simulink model "reactor_test10_sim"  (R2017b)
settings: Solver=ode23tb  StartTime=0.0  StopTime=tEndSimul  MaxStep=0.1  RelTol=5e-6
values from neighbouring files (symbols this model uses):
  c = conversion_factors()    [reactor_test10.m]
  dnDt = 0    [reactor_test10.m]
  h_heater_exterior = 10    [reactor_test10.m]
  h_heater_reactor = 1/R_heater_reactor    (= 400)    [reactor_test10.m]
  qOutIn = 100    [reactor_test10.m]
  Tamb_C = 25    [reactor_test10.m]
  tEnd_dnDt = 0    [reactor_test10.m]
  tEnd_Q = tStart_Q + 120 * c.min_to_sec    [reactor_test10.m]
  Tr_init = param.Tr_init    [reactor_test10.m]
  tStart_dnDt = 0    [reactor_test10.m]
  tStart_Q = 30 * c.min_to_sec    [reactor_test10.m]
undefined symbols (not defined in the file or in its folder): gas, h, liquid, NH3, P, T, T_heater_OFF_C, T_heater_ON_C, tEnd, tStart
libraries: thermochemical x17, simulink x3, dspsigops x1
settings Model: Creator=ferru  LastModifiedBy=fferrucc
settings SolverCC: AlgebraicLoopSolver=LineSearch

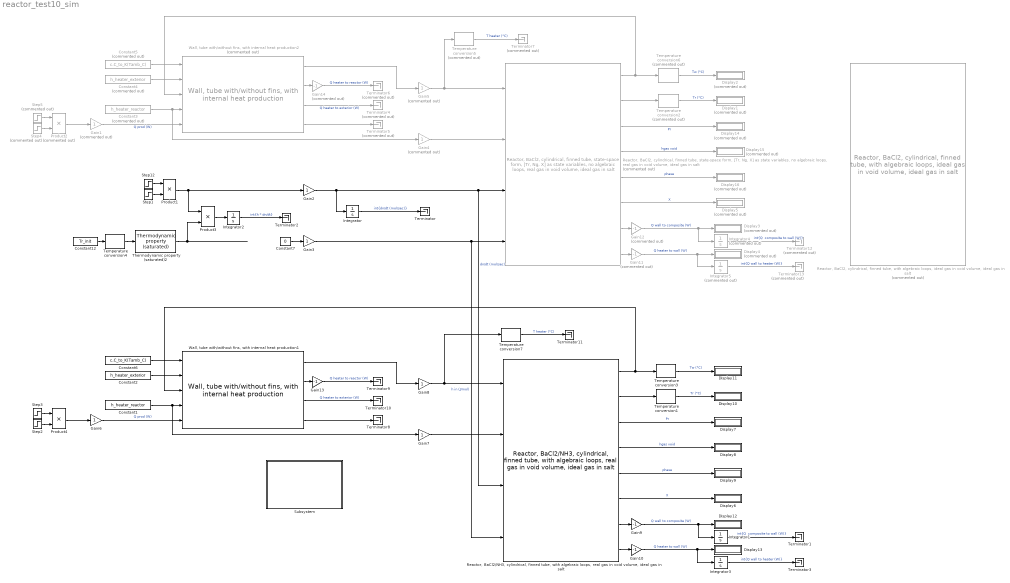
== system reactor_test10_sim ==
  Constant1 : Constant  Value=h_heater_reactor
  Constant12 : Constant  Value=Tr_init
  Constant2 : Constant  Value=h_heater_exterior
  Constant3 : Constant  Commented=on  Value=h_heater_reactor
  Constant4 : Constant  Commented=on  Value=h_heater_exterior
  Constant5 : Constant  Commented=on  Value=c.C_to_K(Tamb_C)
  Constant6 : Constant  Value=c.C_to_K(Tamb_C)
  Constant7 : Constant  Value=0
  Display{1..5,14..16} (8 alike) : Display  Commented=on
  Display{6..13} (8 alike) : Display
  Gain1 : Gain  Commented=on
  Gain10 : Gain  Gain=-1
  Gain11 : Gain  Commented=on  Gain=-1
  Gain12 : Gain  Commented=on  Gain=-1
  Gain13 : Gain  Gain=-1
  Gain14 : Gain  Commented=on  Gain=-1
  Gain{2..3,6..8} (5 alike) : Gain
  Gain4 : Gain  Commented=on
  Gain5 : Gain  Commented=on
  Gain9 : Gain  Gain=-1
  Integrator{,1..3} (4 alike) : Integrator
  Integrator4 : Integrator  Commented=on
  Integrator5 : Integrator  Commented=on
  Product1 : Product
  Product2 : Product  Commented=on
  Product3 : Product
  Product4 : Product
  "Reactor, BaCl2, cylindrical, finned tube, state-space form, [Tr, Ng, X] as state variables, no algebraic loops, real gas in void volume, ideal gas in salt" : thermochemical/Reactors/Reactor, BaCl2//NH3, state-space form, [Tr, Ng, X] as state variables, no algebraic loops, real gas in void volume, ideal gas in salt/Reactor, BaCl2, cylindrical, finned tube, state-space form, [Tr, Ng, X] as state variables, no algebraic loops, real gas in void volume, ideal gas in salt  Commented=on
      link override "Reactor, BaCl2//NH3, cylindrical, no walls, state-space form, [Tr, Ng, X] as state variables, no algebraic loops, real gas in void volume, ideal gas in salt": tao_salt=param.tao_salt  rho_composite=param.rho_composite  K_cin=K_cin  fluid=fluid  Lr=param.Lr  Lr_total=param.Lr_total  Dr=param.D  Ddiff=param.Ddiff  Tr_init=param.Tr_init  X_init=param.X_init
      link override "Wall, tube with//without fins": L_m=param.Lr_total  OD_mm=OD_mm  e_mm=thickness_mm  Tinit=Ttube_init
      settings: SourceProductName=@ Thermochemical
  "Reactor, BaCl2, cylindrical, finned tube, with algebraic loops, ideal gas in void volume, ideal gas in salt" : thermochemical/Reactors/Reactor, BaCl2//NH3, with algebraic loops, ideal gas in void volume, ideal gas in salt/Reactor, BaCl2, cylindrical, finned tube, with algebraic loops, ideal gas in void volume, ideal gas in salt  Commented=on
      link override "Reactor, BaCl2//NH3, cylindrical, no walls, with algebraic loops, ideal gas in void volume, ideal gas in salt": tao_salt=param.tao_salt  rho_composite=param.rho_composite  K_cin=K_cin  fluid=fluid  Lr=param.Lr  Lr_total=param.Lr_total  Dr=param.D  Ddiff=param.Ddiff  Tr_init=param.Tr_init  X_init=param.X_init
      link override "Wall, tube with//without fins": L_m=param.Lr_total  OD_mm=OD_mm  e_mm=thickness_mm  Tinit=Ttube_init
      settings: SourceProductName=@ Thermochemical
  "Reactor, BaCl2/NH3, cylindrical, finned tube, with algebraic loops, real gas in void volume, ideal gas in salt" : thermochemical/Reactors/Reactor, BaCl2//NH3, with algebraic loops, real gas in void volume, ideal gas in salt/Reactor, BaCl2//NH3, cylindrical, finned tube, with algebraic loops, real gas in void volume, ideal gas in salt
      link override "Reactor, BaCl2//NH3, cylindrical, no walls, with algebraic loops, real gas in void volume, ideal gas in salt": tao_salt=param.tao_salt  rho_composite=param.rho_composite  K_cin=K_cin  fluid=fluid  Lr=param.Lr  Lr_total=param.Lr_total  Dr=param.D  Ddiff=param.Ddiff  Tr_init=param.Tr_init  X_init=param.X_init
      link override "Wall, tube with//without fins": L_m=param.Lr_total  OD_mm=OD_mm  e_mm=thickness_mm  Tinit=Ttube_init
      settings: SourceProductName=@ Thermochemical
  Step1 : Step  Time=tEnd_dnDt  Before=1  After=0  SampleTime=0
  Step12 : Step  Time=tStart_dnDt  After=dnDt  SampleTime=0
  Step2 : Step  Time=tEnd_Q  Before=1  After=0  SampleTime=0
  Step3 : Step  Time=tStart_Q  After=qOutIn  SampleTime=0
  Step4 : Step  Commented=on  Time=tEnd_Q  Before=1  After=0  SampleTime=0
  Step5 : Step  Commented=on  Time=tStart_Q  After=qOutIn  SampleTime=0
  Subsystem : Subsystem
  Temperature conversion1 : thermochemical/Conversions/Temperature conversion  sel=K --> °C
      settings: SourceProductName=@ Thermochemical
  Temperature conversion2 : thermochemical/Conversions/Temperature conversion  Commented=on  sel=K --> °C
      settings: SourceProductName=@ Thermochemical
  Temperature conversion3 : thermochemical/Conversions/Temperature conversion  sel=K --> °C
      settings: SourceProductName=@ Thermochemical
  Temperature conversion4 : thermochemical/Conversions/Temperature conversion  sel=°C --> K
      settings: SourceProductName=@ Thermochemical
  Temperature conversion5 : thermochemical/Conversions/Temperature conversion  Commented=on  sel=K --> °C
      settings: SourceProductName=@ Thermochemical
  Temperature conversion6 : thermochemical/Conversions/Temperature conversion  Commented=on  sel=K --> °C
      settings: SourceProductName=@ Thermochemical
  Temperature conversion7 : thermochemical/Conversions/Temperature conversion  sel=K --> °C
      settings: SourceProductName=@ Thermochemical
  Terminator{,1..3,8..11} (8 alike) : Terminator
  Terminator{4..7,12..13} (6 alike) : Terminator  Commented=on
  Thermodynamic property (saturated)2 : thermochemical/Thermodynamic fluid properties/Thermodynamic  property (saturated)  sel=h(T) vap. (J/mol)  fluid=fluid  lookup1D_BreakPoint1=fluid.sat.T  lookup1D_Data=fluid.sat.vap.h_molar
      settings: SourceProductName=@ Thermochemical
  "Wall, tube with/without fins, with internal heat production1" : thermochemical/Walls/Wall, tube with//without fins, with internal heat production  L_m=heater_length_m  OD_mm=heater_OD_mm  e_mm=heater_thickness_mm  material_tube=Steel  cp_tube=464.5  rho_tube=7847  height_fin_mm=0  thickness_fin_mm=0  pitch_fin_mm=0  material_fin=Aluminum 1100  cp_fin=905.9  rho_fin=2658  lambda_fin=211.8  Tinit=Theater_init  mass_tube=2.829  mass_fin=0  mass_total=2.829  s_inner=0.35744  s_outer=0.3636
      settings: SourceProductName=@ Thermochemical
  "Wall, tube with/without fins, with internal heat production2" : thermochemical/Walls/Wall, tube with//without fins, with internal heat production  Commented=on  L_m=heater_length_m  OD_mm=heater_OD_mm  e_mm=heater_thickness_mm  material_tube=Steel  cp_tube=464.5  rho_tube=7847  height_fin_mm=0  thickness_fin_mm=0  pitch_fin_mm=0  material_fin=Aluminum 1100  cp_fin=905.9  rho_fin=2658  lambda_fin=211.8  Tinit=Theater_init  mass_tube=2.829  mass_fin=0  mass_total=2.829  s_inner=0.35744  s_outer=0.3636
      settings: SourceProductName=@ Thermochemical
  wires:
  Gain2/1 -> Integrator/1, "Reactor, BaCl2, cylindrical, finned tube, state-space form, [Tr, Ng, X] as state variables, no algebraic loops, real gas in void volume, ideal gas in salt"/3, "Reactor, BaCl2/NH3, cylindrical, finned tube, with algebraic loops, real gas in void volume, ideal gas in salt"/3  "dn/dt (mol/sec)"
  Gain3/1 -> "Reactor, BaCl2, cylindrical, finned tube, state-space form, [Tr, Ng, X] as state variables, no algebraic loops, real gas in void volume, ideal gas in salt"/4, "Reactor, BaCl2/NH3, cylindrical, finned tube, with algebraic loops, real gas in void volume, ideal gas in salt"/4  "h in (J/mol)"
  "Reactor, BaCl2/NH3, cylindrical, finned tube, with algebraic loops, real gas in void volume, ideal gas in salt"/3 -> Display7/1  "Pr"
  "Reactor, BaCl2/NH3, cylindrical, finned tube, with algebraic loops, real gas in void volume, ideal gas in salt"/4 -> Display8/1  "hgas void"
  "Reactor, BaCl2/NH3, cylindrical, finned tube, with algebraic loops, real gas in void volume, ideal gas in salt"/2 -> Temperature conversion1/1
  "Reactor, BaCl2/NH3, cylindrical, finned tube, with algebraic loops, real gas in void volume, ideal gas in salt"/6 -> Display6/1  "X"
  "Reactor, BaCl2/NH3, cylindrical, finned tube, with algebraic loops, real gas in void volume, ideal gas in salt"/5 -> Display9/1  "phase"
  Product1/1 -> Gain2/1, Product3/1
  Step12/1 -> Product1/1
  Step1/1 -> Product1/2
  Integrator/1 -> Terminator/1  "int{dn/dt (mol/sec)}"
  Integrator1/1 -> Terminator1/1  "int{Q  composite to wall (W)}"
  Temperature conversion1/1 -> Display10/1  "Tr (°C)"
  Constant12/1 -> Temperature conversion4/1
  Thermodynamic property (saturated)2/1 -> Product3/2
  Temperature conversion4/1 -> Thermodynamic property (saturated)2/1
  Integrator2/1 -> Terminator2/1  "int{h * dn/dt}"
  Product3/1 -> Integrator2/1
  Temperature conversion3/1 -> Display11/1  "Tw (°C)"
  "Reactor, BaCl2/NH3, cylindrical, finned tube, with algebraic loops, real gas in void volume, ideal gas in salt"/7 -> Gain9/1
  "Reactor, BaCl2/NH3, cylindrical, finned tube, with algebraic loops, real gas in void volume, ideal gas in salt"/8 -> Gain10/1
  Temperature conversion2/1 -> Display1/1  "Tr (°C)"
  Temperature conversion6/1 -> Display2/1  "Tw (°C)"
  "Reactor, BaCl2, cylindrical, finned tube, state-space form, [Tr, Ng, X] as state variables, no algebraic loops, real gas in void volume, ideal gas in salt"/4 -> Display15/1  "hgas void"
  "Reactor, BaCl2, cylindrical, finned tube, state-space form, [Tr, Ng, X] as state variables, no algebraic loops, real gas in void volume, ideal gas in salt"/5 -> Display16/1  "phase"
  "Reactor, BaCl2, cylindrical, finned tube, state-space form, [Tr, Ng, X] as state variables, no algebraic loops, real gas in void volume, ideal gas in salt"/2 -> Temperature conversion2/1
  "Reactor, BaCl2, cylindrical, finned tube, state-space form, [Tr, Ng, X] as state variables, no algebraic loops, real gas in void volume, ideal gas in salt"/6 -> Display5/1  "X"
  "Reactor, BaCl2, cylindrical, finned tube, state-space form, [Tr, Ng, X] as state variables, no algebraic loops, real gas in void volume, ideal gas in salt"/3 -> Display14/1  "Pr"
  Gain5/1 -> "Reactor, BaCl2, cylindrical, finned tube, state-space form, [Tr, Ng, X] as state variables, no algebraic loops, real gas in void volume, ideal gas in salt"/1, Temperature conversion5/1
  Gain4/1 -> "Reactor, BaCl2, cylindrical, finned tube, state-space form, [Tr, Ng, X] as state variables, no algebraic loops, real gas in void volume, ideal gas in salt"/2
  Integrator3/1 -> Terminator3/1  "int{Q wall to heater (W)}"
  Constant4/1 -> "Wall, tube with/without fins, with internal heat production2"/2
  Constant5/1 -> "Wall, tube with/without fins, with internal heat production2"/1
  Gain1/1 -> "Wall, tube with/without fins, with internal heat production2"/5  "Q prod (W)"
  Step4/1 -> Product2/2
  Step5/1 -> Product2/1
  Product2/1 -> Gain1/1
  Temperature conversion5/1 -> Terminator7/1  "T heater (°C)"
  "Wall, tube with/without fins, with internal heat production2"/1 -> Gain5/1
  Constant3/1 -> "Wall, tube with/without fins, with internal heat production2"/4, Gain4/1
  "Reactor, BaCl2, cylindrical, finned tube, state-space form, [Tr, Ng, X] as state variables, no algebraic loops, real gas in void volume, ideal gas in salt"/1 -> "Wall, tube with/without fins, with internal heat production2"/3, Temperature conversion6/1
  Temperature conversion7/1 -> Terminator11/1  "T heater (°C)"
  "Wall, tube with/without fins, with internal heat production1"/3 -> Terminator10/1  "Q heater to exterior (W)"
  Gain7/1 -> "Reactor, BaCl2/NH3, cylindrical, finned tube, with algebraic loops, real gas in void volume, ideal gas in salt"/2
  Product4/1 -> Gain6/1
  Constant1/1 -> Gain7/1, "Wall, tube with/without fins, with internal heat production1"/4
  "Reactor, BaCl2/NH3, cylindrical, finned tube, with algebraic loops, real gas in void volume, ideal gas in salt"/1 -> "Wall, tube with/without fins, with internal heat production1"/3, Temperature conversion3/1
  Constant2/1 -> "Wall, tube with/without fins, with internal heat production1"/2
  Gain6/1 -> "Wall, tube with/without fins, with internal heat production1"/5  "Q prod (W)"
  "Wall, tube with/without fins, with internal heat production1"/2 -> Gain13/1
  Step3/1 -> Product4/1
  Constant6/1 -> "Wall, tube with/without fins, with internal heat production1"/1
  "Wall, tube with/without fins, with internal heat production1"/4 -> Terminator8/1
  Step2/1 -> Product4/2
  "Wall, tube with/without fins, with internal heat production1"/1 -> Gain8/1
  Gain8/1 -> Temperature conversion7/1, "Reactor, BaCl2/NH3, cylindrical, finned tube, with algebraic loops, real gas in void volume, ideal gas in salt"/1
  Gain9/1 -> Integrator1/1, Display12/1  "Q wall to composite (W)"
  Gain10/1 -> Integrator3/1, Display13/1  "Q heater to wall (W)"
  Gain11/1 -> Integrator5/1, Display4/1  "Q heater to wall (W)"
  "Reactor, BaCl2, cylindrical, finned tube, state-space form, [Tr, Ng, X] as state variables, no algebraic loops, real gas in void volume, ideal gas in salt"/8 -> Gain11/1
  Integrator4/1 -> Terminator12/1  "int{Q  composite to wall (W)}"
  Gain12/1 -> Integrator4/1, Display3/1  "Q wall to composite (W)"
  Integrator5/1 -> Terminator13/1  "int{Q wall to heater (W)}"
  "Reactor, BaCl2, cylindrical, finned tube, state-space form, [Tr, Ng, X] as state variables, no algebraic loops, real gas in void volume, ideal gas in salt"/7 -> Gain12/1
  Gain13/1 -> Terminator9/1  "Q heater to reactor (W)"
  "Wall, tube with/without fins, with internal heat production2"/4 -> Terminator5/1
  "Wall, tube with/without fins, with internal heat production2"/3 -> Terminator4/1  "Q heater to exterior (W)"
  "Wall, tube with/without fins, with internal heat production2"/2 -> Gain14/1
  Gain14/1 -> Terminator6/1  "Q heater to reactor (W)"
  Constant7/1 -> Gain3/1

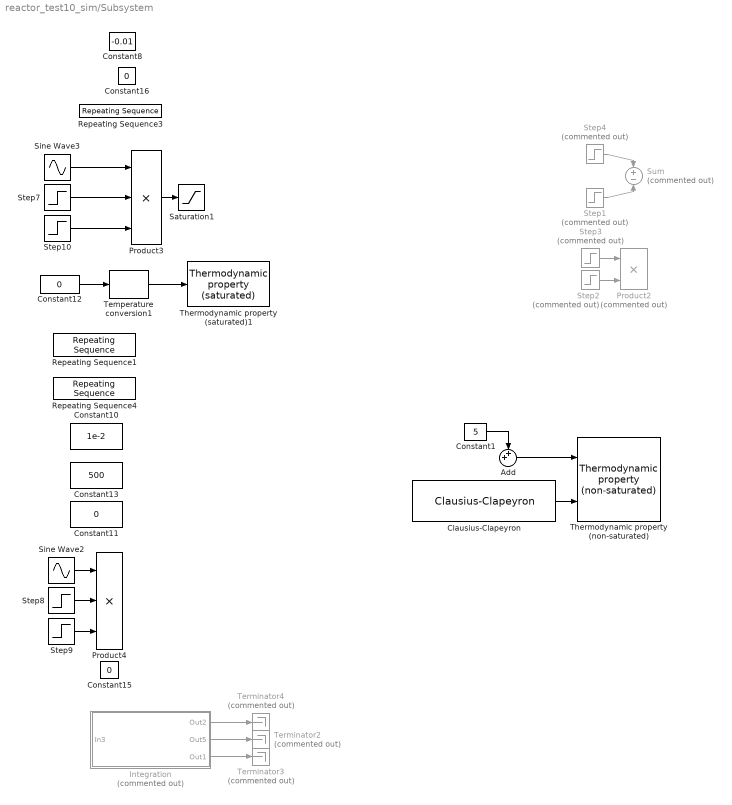
== system reactor_test10_sim/Subsystem ==
  Add : Sum  Inputs=++|
  Clausius-Clapeyron : thermochemical/Thermodynamic fluid properties/Clausius-Clapeyron  sel_1=P(T)  sel_2=NH3(liquid)/NH3(gas)
      settings: SourceProductName=@ Thermochemical
  Constant1 : Constant  Value=5
  Constant10 : Constant  Value=1e-2
  Constant{11..12,15..16} (4 alike) : Constant  Value=0
  Constant13 : Constant  Value=500
  Constant8 : Constant  Value=-0.01
  Integration : Subsystem  Commented=on  mask{T1=tStart, T2=tEnd}
      mask prompts: T1 "Integration time window, start time (sec)"; T2 "Integration time window, stop time (sec)"
  Product2 : Product  Commented=on
  Product3 : Product  Inputs=3
  Product4 : Product  Inputs=3
  Repeating Sequence1 : simulink/Sources/Repeating Sequence  rep_seq_t=[0, 100, 101, 200, 201]  rep_seq_y=[0, 0, 0.01, 0.01, 0]
  Repeating Sequence3 : simulink/Sources/Repeating Sequence  rep_seq_t=[0, 1, 1.001, 1.1, 1.1001, 1.2, 1.2002, 1.3, 1.3001]*1e3  rep_seq_y=[0, 0, 1, 1, 0, 0, 1, 1, 0]*(-0.01)
  Repeating Sequence4 : simulink/Sources/Repeating Sequence  rep_seq_t=[0, 99, 100, 199, 200 299]  rep_seq_y=1000*[0, 0, 1, 1, -1, -1]
  Saturation1 : Saturate  UpperLimit=Inf  LowerLimit=0
  Sine Wave2 : Sin  Amplitude=1e3  Frequency=2*pi/1e2  SampleTime=0
  Sine Wave3 : Sin  Amplitude=0.01  Bias=0.01  Frequency=2*pi/1e2  SampleTime=0
  Step1 : Step  Commented=on  Time=tEnd  After=T_heater_ON_C-T_heater_OFF_C  SampleTime=0
  Step10 : Step  Time=2e3  Before=1  After=0  SampleTime=0
  Step2 : Step  Commented=on  Time=tEnd  Before=1  After=0  SampleTime=0
  Step3 : Step  Commented=on  Time=tStart  After=qOutIn  SampleTime=0
  Step4 : Step  Commented=on  Time=tStart  Before=T_heater_OFF_C  After=T_heater_ON_C  SampleTime=0
  Step7 : Step  Time=1e3  SampleTime=0
  Step8 : Step  Time=1e3  SampleTime=0
  Step9 : Step  Time=2e3  Before=1  After=0  SampleTime=0
  Sum : Sum  Commented=on  Inputs=+-
  Temperature conversion1 : thermochemical/Conversions/Temperature conversion  sel=°R --> °F
      settings: SourceProductName=@ Thermochemical
  Terminator2 : Terminator  Commented=on
  Terminator3 : Terminator  Commented=on
  Terminator4 : Terminator  Commented=on
  Thermodynamic property (non-saturated) : thermochemical/Thermodynamic fluid properties/Thermodynamic  property (non-saturated)  sel=h(T,P)  fluid=fluid  reciprocVar=-1  lookup2D_BreakPoint1=fluid.no_sat.T_P_indep.var_indep.T  lookup2D_BreakPoint2=fluid.no_sat.T_P_indep.var_indep.P  lookup2D_Data=fluid.no_sat.T_P_indep.var_dep.h_molar
      settings: SourceProductName=@ Thermochemical
  Thermodynamic property (saturated)1 : thermochemical/Thermodynamic fluid properties/Thermodynamic  property (saturated)  sel=h(T) vap. (J/mol)  fluid=fluid  lookup1D_BreakPoint1=fluid.sat.T  lookup1D_Data=fluid.sat.vap.h_molar
      settings: SourceProductName=@ Thermochemical
  wires:
  Step7/1 -> Product3/2
  Product3/1 -> Saturation1/1
  Sine Wave2/1 -> Product4/1
  Sine Wave3/1 -> Product3/1
  Step8/1 -> Product4/2
  Step10/1 -> Product3/3
  Step9/1 -> Product4/3
  Temperature conversion1/1 -> Thermodynamic property (saturated)1/1
  Constant12/1 -> Temperature conversion1/1
  Integration/2(Out5) -> Terminator2/1
  Integration/3(Out1) -> Terminator3/1
  Integration/1(Out2) -> Terminator4/1
  Add/1 -> Thermodynamic property (non-saturated)/1
  Constant1/1 -> Add/1
  Clausius-Clapeyron/1 -> Thermodynamic property (non-saturated)/2
  ? -> Clausius-Clapeyron/1, Add/2
  Step3/1 -> Product2/1
  Step2/1 -> Product2/2
  Step4/1 -> Sum/1
  Step1/1 -> Sum/2

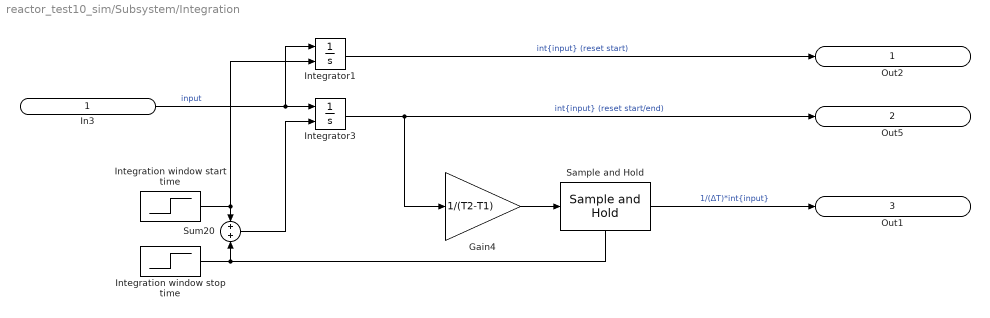
== system reactor_test10_sim/Subsystem/Integration ==
  In3 : Inport
  Gain4 : Gain  Gain=1/(T2-T1)
  Integration window start time : Step  Time=T1  Before=1  After=0  SampleTime=0
  Integration window stop time : Step  Time=T2  SampleTime=0
  Integrator1 : Integrator  ExternalReset=level hold
  Integrator3 : Integrator  ExternalReset=level hold
  Sample and Hold : dspsigops/Sample and Hold  trig=Rising edge  initCond=0  latchinput=on
  Sum20 : Sum
  Out2 : Outport
  Out5 : Outport  Port=2
  Out1 : Outport  Port=3
  wires:
  Sample and Hold/1 -> Out1/1  "1/(ΔT)*int{input}"
  Gain4/1 -> Sample and Hold/1
  Sum20/1 -> Integrator3/2
  In3/1 -> Integrator1/1, Integrator3/1  "input"
  Integrator3/1 -> Out5/1, Gain4/1  "int{input} (reset start/end)"
  Integration window start time/1 -> Integrator1/2, Sum20/1
  Integration window stop time/1 -> Sum20/2, Sample and Hold/Trigger
  Integrator1/1 -> Out2/1  "int{input} (reset start)"
